simulink model "ReceivingMachine"  (R2016b)
settings: Solver=FixedStepAuto  StartTime=0.0  StopTime=10.0  RelTol=1e-3
undefined symbols (not defined in the file): MotorSpeed
settings Model: Creator=NEATdemo  LastModifiedBy=NEATdemo

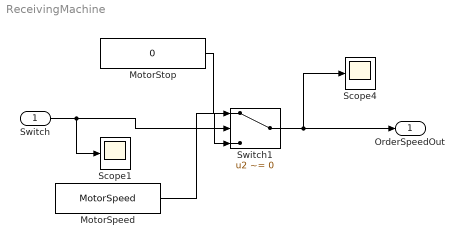
== system ReceivingMachine ==
  Switch : Inport
  MotorSpeed : Constant  Value=MotorSpeed
  MotorStop : Constant  Value=0
  Scope1 : Scope
  Scope4 : Scope
  Switch1 : Switch  Criteria=u2 ~= 0  Threshold=1
  OrderSpeedOut : Outport
      settings: AttributesFormatString=speed
  wires:
  Switch/1 -> Scope1/1, Switch1/2
  MotorStop/1 -> Switch1/3
  MotorSpeed/1 -> Switch1/1
  Switch1/1 -> Scope4/1, OrderSpeedOut/1
